simulink model "DOYLIA"  (R2019b)
settings: Solver=VariableStepAuto  StartTime=0.0  StopTime=9*3600  RelTol=1e-3
undefined symbols (not defined in the file or in its folder): m, n, TimeOut, TimeOut1, TimeOut2, TimeQuene, TimeQuene1, TimeServer1, TimeServer2
libraries: simulink x2
settings Model: Creator=Εμμανουήλ  LastModifiedBy=Εμμανουήλ
settings DataIOCC: Decimation=10  Refine=10
settings OptimizationCC: UseDivisionForNetSlopeComputation=on
settings RTWCC: GenCodeOnly=on

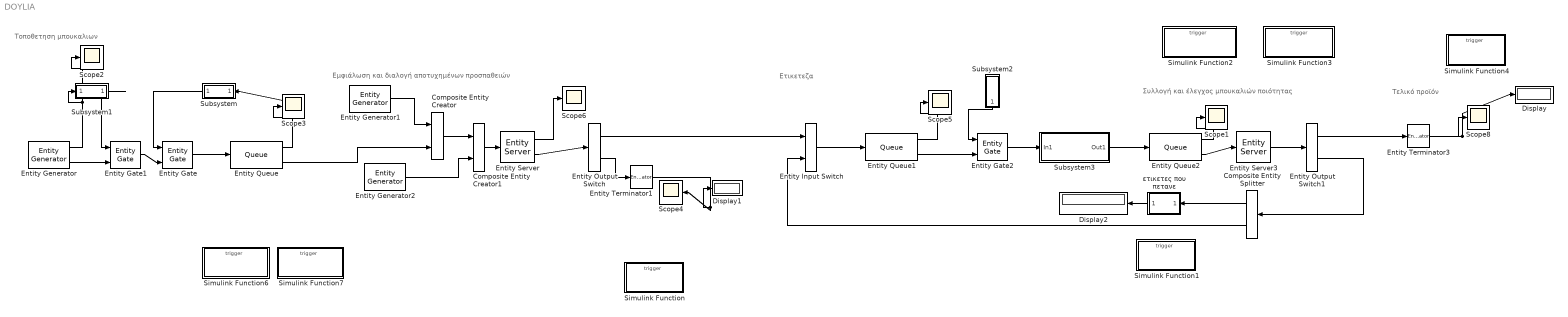
== system DOYLIA ==
  note: Τελικό προϊόν
  note: Συλλογή και έλεγχος μπουκαλιών ποιότητας
  note: Ετικετεζα
  note: Εμφιάλωση και διαλογή αποτυχημένων προσπαθειών
  note: Τοποθετηση μπουκαλιων
  Composite Entity Creator : CompositeEntityCreator  InputPortMessageModes=m,m  OutputPortMessageModes=m  EntityTypeName=Water  InputEntityName=W1|W2
      settings: InputPortMap=u0,u1
  Composite Entity Creator1 : CompositeEntityCreator  InputPortMessageModes=m,m  OutputPortMessageModes=m  EntityTypeName=Cap  InputEntityName=C1|C2
      settings: InputPortMap=u0,u1
  Composite Entity Splitter : CompositeEntitySplitter  InputPortMessageModes=m  OutputPortMessageModes=m,m
      settings: OutputPortMap=o0,o1
  Display : Display
  Display1 : Display
  Display2 : Display
  Entity Input Switch : EntityInputSwitch  InputPortMessageModes=m,m  OutputPortMessageModes=m
  Entity Output Switch : EntityOutputSwitch  InputPortMessageModes=m  OutputPortMessageModes=m,m  SwitchingCriterion=From attribute  SwitchAttributeName=C1.W1.data
  Entity Output Switch1 : EntityOutputSwitch  InputPortMessageModes=m  OutputPortMessageModes=m,m  SwitchingCriterion=From attribute  SwitchAttributeName=CA1.cart
  Entity Gate : EntityGate  InputPortMessageModes=m,m  OutputPortMessageModes=m
  Entity Gate1 : EntityGate  InputPortMessageModes=m,m  OutputPortMessageModes=m
  Entity Gate2 : EntityGate  InputPortMessageModes=m,m  OutputPortMessageModes=m
  Entity Generator : EntityGenerator  OutputPortMessageModes=n,m  Period=.5  AttributeName=S1|S2|data3|data4|data5  AttributeInitialValue=1|1|1|1|1  NumberEntitiesDeparted=on  EntityType=Structured  EntityTypeName=Entity
      settings: OutputPortMap=o0,o3
  Entity Generator1 : EntityGenerator  OutputPortMessageModes=m  Period=.5  AttributeName=data  EntityType=Structured  EntityTypeName=WATER
  Entity Generator2 : EntityGenerator  OutputPortMessageModes=m  Period=.5  AttributeName=data1  EntityType=Structured  EntityTypeName=CAP
  Entity Queue : Queue  InputPortMessageModes=m  OutputPortMessageModes=n,m  Capacity=inf  EntryAction=TimeQuene();  ExitAction=TimeQuene1();  NumberEntitiesInBlock=on
      settings: OutputPortMap=o1,o5
  Entity Queue1 : Queue  InputPortMessageModes=m  OutputPortMessageModes=n,m  Capacity=inf  NumberEntitiesInBlock=on
      settings: OutputPortMap=o1,o5
  Entity Queue2 : Queue  InputPortMessageModes=m  OutputPortMessageModes=n,m  Capacity=inf  NumberEntitiesInBlock=on
      settings: OutputPortMap=o1,o5
  Entity Server : EntityServer  InputPortMessageModes=m  OutputPortMessageModes=n,m  Capacity=1  ServiceTimeValue=2  EntryAction=|  WriteResidualTimeToAttribute=on  NumberEntitiesDeparted=on
      | %entity = double;
      | entity.C1.W1.data = randi([1 10000],1,1);
      | 
      | 
      | if (entity.C1.W1.data>=1 && entity.C1.W1.data<=10)
      |     
      |     entity.C1.W1.data = 2;
      | else
      | 
      |     entity.C1.W1.data = 1;
      | end
      settings: OutputPortMap=o0,o9
  Entity Server3 : EntityServer  InputPortMessageModes=m  OutputPortMessageModes=m  Capacity=1  ServiceTimeSource=MATLAB action  ServiceTimeValue=1  ServiceTimeAction=|  EntryAction=TimeServer1();  ExitAction=TimeServer2();
      | persistent rngInit;
      | if isempty(rngInit)
      |     seed = 12345;
      |     rng(seed);
      |     rngInit = true;
      | end
      | 
      | % Pattern: Gaussian (normal) distribution
      | % m: Mean, d: Standard deviation
      | m = 1.5; d = .2;
      | dt = m + d * randn;
  Entity Terminator1 : EntityTerminator  InputPortMessageModes=m  EntryAction=TimeOut();  NumberEntitiesArrived=on
      settings: OutputPortMap=o0
  Entity Terminator3 : EntityTerminator  InputPortMessageModes=m  EntryAction=TimeOut2();  NumberEntitiesArrived=on
      settings: OutputPortMap=o0
  Scope{1..6,8} (7 alike) : Scope
  Simulink Function : Subsystem  TreatAsAtomicUnit=on
  Simulink Function1 : Subsystem  TreatAsAtomicUnit=on
  Simulink Function2 : Subsystem  TreatAsAtomicUnit=on
  Simulink Function3 : Subsystem  TreatAsAtomicUnit=on
  Simulink Function4 : Subsystem  TreatAsAtomicUnit=on
  Simulink Function6 : Subsystem  TreatAsAtomicUnit=on
  Simulink Function7 : Subsystem  TreatAsAtomicUnit=on
  Subsystem : Subsystem
  Subsystem1 : Subsystem
  Subsystem2 : Subsystem
  Subsystem3 : Subsystem
  ετικετες που πετανε : Subsystem
  wires:
  Entity Output Switch/2 -> Entity Terminator1/1
  Entity Queue/2 -> Composite Entity Creator/2
  Entity Queue/1 -> Scope3/1, Subsystem/1(In1)
  Entity Gate/1 -> Entity Queue/1
  Subsystem/1(Out1) -> Entity Gate/1
  Entity Terminator1/1 -> Scope4/1, Display1/1
  Entity Generator/2 -> Entity Gate1/2
  Entity Gate1/1 -> Entity Gate/2
  Subsystem1/1(Out1) -> Entity Gate1/1
  Entity Terminator3/1 -> Display/1, Scope8/1
  Entity Queue2/2 -> Entity Server3/1
  Entity Output Switch1/1 -> Entity Terminator3/1
  Entity Generator/1 -> Scope2/1, Subsystem1/1(In1)
  Entity Gate2/1 -> Subsystem3/1(In1)
  Subsystem2/1(Out1) -> Entity Gate2/1
  Entity Queue1/2 -> Entity Gate2/2
  Entity Queue1/1 -> Scope5/1
  Entity Queue2/1 -> Scope1/1
  Subsystem3/1(Out1) -> Entity Queue2/1
  Entity Generator1/1 -> Composite Entity Creator/1
  Entity Server/2 -> Entity Output Switch/1
  Composite Entity Creator/1 -> Composite Entity Creator1/1
  Composite Entity Creator1/1 -> Entity Server/1
  Entity Generator2/1 -> Composite Entity Creator1/2
  Entity Output Switch/1 -> Entity Input Switch/1
  Entity Input Switch/1 -> Entity Queue1/1
  Entity Server3/1 -> Entity Output Switch1/1
  Entity Output Switch1/2 -> Composite Entity Splitter/1
  Composite Entity Splitter/2 -> Entity Input Switch/2
  Composite Entity Splitter/1 -> ετικετες που πετανε/1(In1)
  ετικετες που πετανε/1(Out1) -> Display2/1
  Entity Server/1 -> Scope6/1

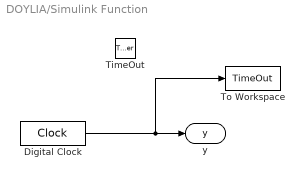
== system DOYLIA/Simulink Function ==
  TimeOut : TriggerPort  TriggerType=function-call  IsSimulinkFunction=on  FunctionName=TimeOut  Variant=on  VariantControl=(inherit)
  Digital Clock : DigitalClock  SampleTime=-1
  To Workspace : ToWorkspace  VariableName=TimeOut  SampleTime=-1
      settings: Save2DSignal=2-D array (concatenate along first dimension)
  y : ArgOut  DisableCoverage=on  ArgumentName=y
  wires:
  Digital Clock/1 -> To Workspace/1, y/1

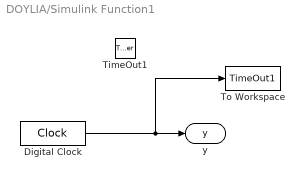
== system DOYLIA/Simulink Function1 ==
  TimeOut1 : TriggerPort  TriggerType=function-call  IsSimulinkFunction=on  FunctionName=TimeOut1  Variant=on  VariantControl=(inherit)
  Digital Clock : DigitalClock  SampleTime=-1
  To Workspace : ToWorkspace  VariableName=TimeOut1  SampleTime=-1
      settings: Save2DSignal=2-D array (concatenate along first dimension)
  y : ArgOut  DisableCoverage=on  ArgumentName=y
  wires:
  Digital Clock/1 -> y/1, To Workspace/1

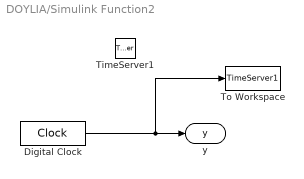
== system DOYLIA/Simulink Function2 ==
  TimeServer1 : TriggerPort  TriggerType=function-call  IsSimulinkFunction=on  FunctionName=TimeServer1  Variant=on  VariantControl=(inherit)
  Digital Clock : DigitalClock  SampleTime=-1
  To Workspace : ToWorkspace  VariableName=TimeServer1  SampleTime=-1
      settings: Save2DSignal=2-D array (concatenate along first dimension)
  y : ArgOut  DisableCoverage=on  ArgumentName=y
  wires:
  Digital Clock/1 -> To Workspace/1, y/1

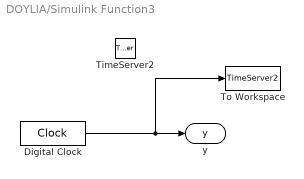
== system DOYLIA/Simulink Function3 ==
  TimeServer2 : TriggerPort  TriggerType=function-call  IsSimulinkFunction=on  FunctionName=TimeServer2  Variant=on  VariantControl=(inherit)
  Digital Clock : DigitalClock  SampleTime=-1
  To Workspace : ToWorkspace  VariableName=TimeServer2  SampleTime=-1
      settings: Save2DSignal=2-D array (concatenate along first dimension)
  y : ArgOut  DisableCoverage=on  ArgumentName=y
  wires:
  Digital Clock/1 -> To Workspace/1, y/1

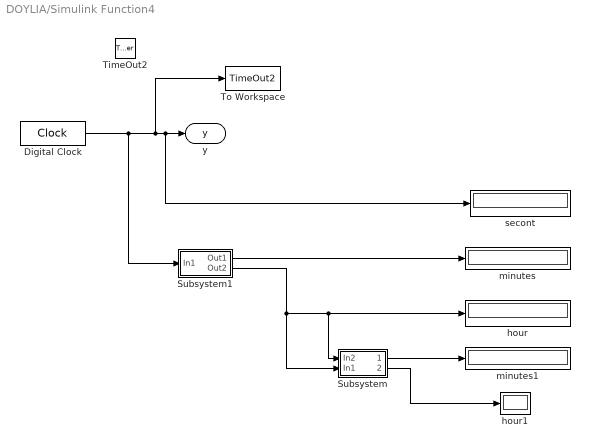
== system DOYLIA/Simulink Function4 ==
  TimeOut2 : TriggerPort  TriggerType=function-call  IsSimulinkFunction=on  FunctionName=TimeOut2  Variant=on  VariantControl=(inherit)
  Digital Clock : DigitalClock  SampleTime=-1
  Subsystem : Subsystem
  Subsystem1 : Subsystem
  To Workspace : ToWorkspace  VariableName=TimeOut2  SampleTime=-1
      settings: Save2DSignal=2-D array (concatenate along first dimension)
  hour : Display
  hour1 : Display
  minutes : Display
  minutes1 : Display
  secont : Display
  y : ArgOut  DisableCoverage=on  ArgumentName=y
  wires:
  Digital Clock/1 -> Subsystem1/1(In1), To Workspace/1, secont/1, y/1
  Subsystem/1(Out1) -> minutes1/1
  Subsystem/2(Out2) -> hour1/1
  Subsystem1/2(Out2) -> Subsystem/2(In1), hour/1, Subsystem/1(In2)
  Subsystem1/1(Out1) -> minutes/1

== system DOYLIA/Simulink Function6 ==
  TimeQuene : TriggerPort  TriggerType=function-call  IsSimulinkFunction=on  FunctionName=TimeQuene  Variant=on  VariantControl=(inherit)
  Digital Clock : DigitalClock  SampleTime=-1
  To Workspace : ToWorkspace  VariableName=TimeQuene  SampleTime=-1
      settings: Save2DSignal=2-D array (concatenate along first dimension)
  y : ArgOut  DisableCoverage=on  ArgumentName=y
  wires:
  Digital Clock/1 -> To Workspace/1, y/1

== system DOYLIA/Simulink Function7 ==
  TimeQuene1 : TriggerPort  TriggerType=function-call  IsSimulinkFunction=on  FunctionName=TimeQuene1  Variant=on  VariantControl=(inherit)
  Digital Clock : DigitalClock  SampleTime=-1
  To Workspace : ToWorkspace  VariableName=TimeQuene1  SampleTime=-1
      settings: Save2DSignal=2-D array (concatenate along first dimension)
  y : ArgOut  DisableCoverage=on  ArgumentName=y
  wires:
  Digital Clock/1 -> y/1, To Workspace/1

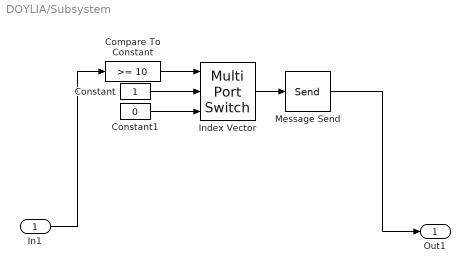
== system DOYLIA/Subsystem ==
  In1 : Inport
  Compare To Constant : simulink/Logic and Bit Operations/Compare To Constant  relop=>=  const=10  OutDataTypeStr=boolean
  Constant : Constant
  Constant1 : Constant  Value=0
  Index Vector : MultiPortSwitch  DataPortOrder=Zero-based contiguous  Inputs=2  zeroidx=on
  Message Send : Send  OutputPortMessageModes=m
  Out1 : Outport
  wires:
  Constant1/1 -> Index Vector/3
  Constant/1 -> Index Vector/2
  Index Vector/1 -> Message Send/1
  In1/1 -> Compare To Constant/1
  Compare To Constant/1 -> Index Vector/1
  Message Send/1 -> Out1/1

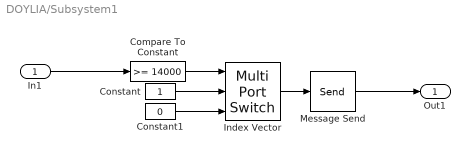
== system DOYLIA/Subsystem1 ==
  In1 : Inport
  Compare To Constant : simulink/Logic and Bit Operations/Compare To Constant  relop=>=  const=14000  OutDataTypeStr=boolean
  Constant : Constant
  Constant1 : Constant  Value=0
  Index Vector : MultiPortSwitch  DataPortOrder=Zero-based contiguous  Inputs=2  zeroidx=on
  Message Send : Send  OutputPortMessageModes=m
  Out1 : Outport
  wires:
  Message Send/1 -> Out1/1
  Compare To Constant/1 -> Index Vector/1
  In1/1 -> Compare To Constant/1
  Index Vector/1 -> Message Send/1
  Constant/1 -> Index Vector/2
  Constant1/1 -> Index Vector/3

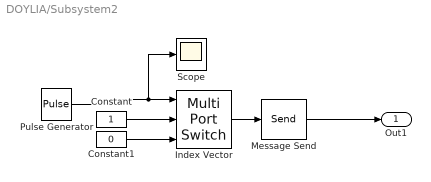
== system DOYLIA/Subsystem2 ==
  Constant : Constant
  Constant1 : Constant  Value=0
  Index Vector : MultiPortSwitch  DataPortOrder=Zero-based contiguous  Inputs=2  zeroidx=on
  Message Send : Send  OutputPortMessageModes=m
  Pulse Generator : DiscretePulseGenerator  PulseType=Time based  Period=2020  PulseWidth=1.5
  Scope : Scope
  Out1 : Outport
  wires:
  Message Send/1 -> Out1/1
  Index Vector/1 -> Message Send/1
  Constant/1 -> Index Vector/2
  Constant1/1 -> Index Vector/3
  Pulse Generator/1 -> Scope/1, Index Vector/1

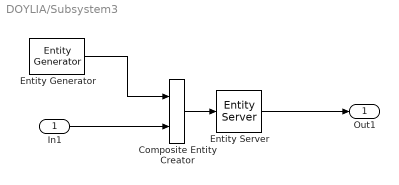
== system DOYLIA/Subsystem3 ==
  In1 : Inport
  Composite Entity Creator : CompositeEntityCreator  InputPortMessageModes=m,m  OutputPortMessageModes=m  EntityTypeName=CART1  InputEntityName=CA1|CA2
      settings: InputPortMap=u0,u1
  Entity Generator : EntityGenerator  OutputPortMessageModes=m  Period=.5  AttributeName=cart  EntityType=Structured  EntityTypeName=CART
  Entity Server : EntityServer  InputPortMessageModes=m  OutputPortMessageModes=m  Capacity=1  ServiceTimeValue=1  EntryAction=|
      | entity.CA1.cart = randi([1 1000],1,1);
      | 
      | if (entity.CA1.cart>=1 && entity.CA1.cart<=20)
      |     
      |    entity.CA1.cart = 2;
      | else
      |     
      |     entity.CA1.cart = 1;
      | end
  Out1 : Outport
  wires:
  Entity Server/1 -> Out1/1
  In1/1 -> Composite Entity Creator/2
  Entity Generator/1 -> Composite Entity Creator/1
  Composite Entity Creator/1 -> Entity Server/1

== system DOYLIA/ετικετες που πετανε ==
  In1 : Inport
  Entity Terminator2 : EntityTerminator  InputPortMessageModes=m  EntryAction=TimeOut1();  NumberEntitiesArrived=on
      settings: OutputPortMap=o0
  Scope6 : Scope
  Out1 : Outport
  wires:
  Entity Terminator2/1 -> Out1/1, Scope6/1
  In1/1 -> Entity Terminator2/1

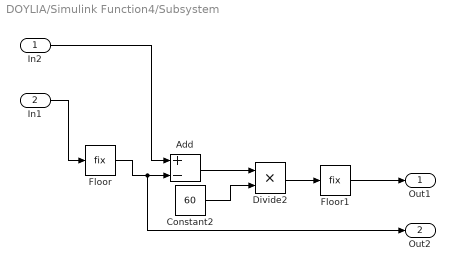
== system DOYLIA/Simulink Function4/Subsystem ==
  In2 : Inport
  In1 : Inport  Port=2
  Add : Sum  Inputs=+-
  Constant2 : Constant  Value=60
  Divide2 : Product  Inputs=**
  Floor : Rounding  Operator=fix
  Floor1 : Rounding  Operator=fix
  Out1 : Outport
  Out2 : Outport  Port=2
  wires:
  Constant2/1 -> Divide2/2
  Floor/1 -> Out2/1, Add/2
  Divide2/1 -> Floor1/1
  Add/1 -> Divide2/1
  In1/1 -> Floor/1
  In2/1 -> Add/1
  Floor1/1 -> Out1/1

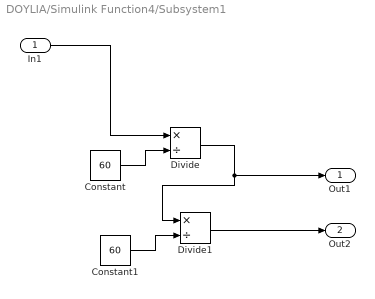
== system DOYLIA/Simulink Function4/Subsystem1 ==
  In1 : Inport
  Constant : Constant  Value=60
  Constant1 : Constant  Value=60
  Divide : Product  Inputs=*/
  Divide1 : Product  Inputs=*/
  Out1 : Outport
  Out2 : Outport  Port=2
  wires:
  Constant/1 -> Divide/2
  Divide/1 -> Out1/1, Divide1/1
  Divide1/1 -> Out2/1
  Constant1/1 -> Divide1/2
  In1/1 -> Divide/1
